simulink model "RELAY_TUNING"  (R2021a)
settings: Solver=VariableStepAuto  StartTime=0.0  StopTime=15.0  RelTol=1e-3
values from neighbouring files (symbols this model uses):
  K = 1.5286    [Q2_RELAY.m]
  tau = 0.0254    [Q2_RELAY.m]
settings Model: Creator=Doron and Sagit  LastModifiedBy=Doron and Sagit

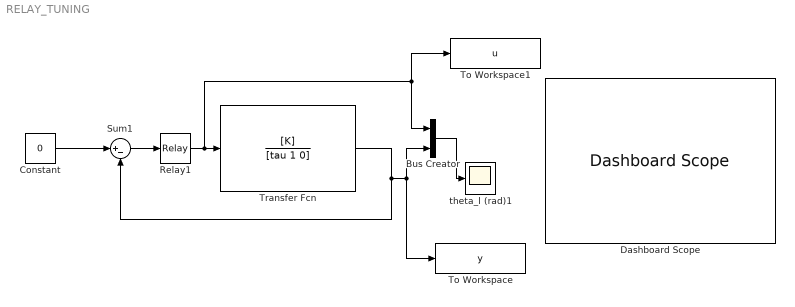
== system RELAY_TUNING ==
  Bus Creator : BusCreator  Inputs=2
  Constant : Constant  Value=0
  Dashboard Scope : DashboardScope
  Relay1 : Relay  OnSwitchValue=0.1  OffSwitchValue=-0.1  OffOutputValue=-1
  Sum1 : Sum  Inputs=|+-
  To Workspace : ToWorkspace  VariableName=y  SampleTime=-1
  To Workspace1 : ToWorkspace  VariableName=u  SampleTime=-1
  Transfer Fcn : TransferFcn  Numerator=[K]  Denominator=[tau 1 0]
  theta_l (rad)1 : Scope
  wires:
  Transfer Fcn/1 -> Bus Creator/2, To Workspace/1, Sum1/2
  Sum1/1 -> Relay1/1
  Constant/1 -> Sum1/1
  Relay1/1 -> To Workspace1/1, Bus Creator/1, Transfer Fcn/1
  Bus Creator/1 -> theta_l (rad)1/1
